simulink model "blocks"  (Simulink 6.6)
settings: Solver=FixedStepDiscrete  StartTime=0.0  StopTime=10.0  FixedStep=0.001  RelTol=1e-3
undefined symbols (not defined in the file or in its folder): ecan1_init, init_DMA0, init_DMA2, u1
libraries: simulink x11, dsPICdrivers x3
settings Model: Creator=bwmairs  LastModifiedBy=bwmairs  ProdHWDeviceType=16-bit Generic
settings OptimizationCC: InlineParams=on  OptimizeModelRefInitCode=on  LifeSpan=1
settings HardwareCC: ProdBitPerInt=16  ProdEndianess=LittleEndian  ProdWordSize=16  ProdHWDeviceType=16-bit Generic  TargetHWDeviceType=32-bit Generic
settings RTWCC: SystemTargetFile=dspic.tlc  TemplateMakefile=dspic_pic30_gcc.tmf  PostCodeGenCommand=dsPIC_Compile()  Description=Embedded Target for Microchip dsPIC (real-time)  ProcessScript=dspic_make_rtw_hook
settings CodeAppCC: IgnoreCustomStorageClasses=off
settings STFCustomTargetCC: TargetFcnLib=ansi_tfl_tmw.mat  GenFloatMathFcnCalls=ANSI_C  ModelReferenceCompliant=off  IncludeMdlTerminateFcn=off  CombineOutputUpdateFcns=on  SuppressErrorStatus=on  ERTCustomFileBanners=on  SupportContinuousTime=off  SupportNonInlinedSFcns=off  SystemTargetFile=dspic.tlc
settings ERTTargetCC: TargetFcnLib=ansi_tfl_tmw.mat  GenFloatMathFcnCalls=ANSI_C  ModelReferenceCompliant=off  IncludeMdlTerminateFcn=off  SuppressErrorStatus=on  ModelStepFunctionPrototypeControlCompliant=off  InlinedParameterPlacement=NonHierarchical  ERTSrcFileBannerTemplate=dsPIC_code_template.cgt  ERTHdrFileBannerTemplate=dsPIC_code_template.cgt  ERTDataSrcFileTemplate=dsPIC_code_template.cgt  ERTDataHdrFileTemplate=dsPIC_code_template.cgt  ERTCustomFileTemplate=dsPIC_main.tlc
settings CustomProperty: DataType=string  Value=C:\PROGRA~1\MATLAB\R2007a\rtw\bin\win32\gmake

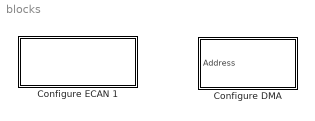
== system blocks ==
  Configure DMA : Subsystem  mask{channel=0, direction=Read, irqsel=INT0, peripheral=0, a_mode=Peripheral Indirect, mode=Continuous, half=when half of data has been moved, nullw=Null data write to peripheral, data_size=Word, batch_size=0}
      mask prompts: channel "DMA Channel"; irqsel "IRQ"; a_mode "Addressing Mode"; half "Trigger Block Transfer Interrupt"; nullw "Null Data Peripheral Write Mode"; data_size "Data Size"; batch_size "Batch Size"
      mask help: CURRENTLY HARDWIRED TO CONFIGURE DMA0!
      mask Help: Batch size - This refers to the DMAxCNT register. It consists of a 10-bit number that is 1 less than the number of requests the channel must service before the data block transfer is considered complete.
      mask StyleString: popup(0|1|2|3|4|5|6|7),popup(Read|Write),popup(INT0|IC1|OC1|IC2|OC2|TMR2|TMR3|SPI1|UART1RX|UART1TX|ADC1|ADC2|UART2RX|UART2TX|SPI2|ECAN1|ECAN2|DCI|ECAN1|ECAN2),edit,popup(Peripheral Indirect|Register Indirect|Register Indirect: Post-Increment),popup(Continuous|One-Shot|Continuous w/ Ping-Pong|One-Shot w/ Ping-Pong),popup(when half of data has been moved|when all the data has been moved),popup(Null data write to peripheral|Normal operation),popup(Word|Byte),edit
      mask Display: text(0.5,0.5,sprintf('Configure DMA%d',str2num(get_param(gcb,'channel'))),'horizontalAlignment','center','verticalAlignment','middle');
  Configure ECAN 1 : Subsystem  mask(Initialize ECAN 1){frame_setting=off, mode=--, dma_rx_chan=0, dma_tx_chan=0, baud=0, ps1=0, pd=0, ps2=0, tq=0, dma_buf_size=4 buffers, rx_bufs=[], tx_bufs=[], buf_0_tx_pri=Highest, buf_1_tx_pri=Lowest, mask_0=0, mask_0_rm=0, mask_1=0, mask_1_rm=0, mask_2=0, mask_2_rm=0, filters=[], filter_0=0, filter_0_mask=0, filter_0_exide=0, filter_0_buf=0, filter_1=0, filter_1_mask=0, filter_1_exide=0, filter_1_buf=0}
      mask prompts: frame_setting "Extended Frames (Standard if unchecked)"; dma_rx_chan "DMA Reception Channel"; dma_tx_chan "DMA Transmission Channel"; baud "Baud Rate"; ps1 "Phase Segment 1"; pd "Propagation Delay"; ps2 "Phase Segment 2"; tq "Time Quanta"; dma_buf_size "DMA Buffer Size"; rx_bufs "Reception Buffers"; tx_bufs "Transmission Buffers"; buf_0_tx_pri "Buffer 0 Transmission Priority"; buf_1_tx_pri "Buffer 1 Transmission Priority"; mask_0 "Mask 0"; mask_0_rm "Mask 0 Receive Mode"; mask_1 "Mask 1"; mask_1_rm "Mask 1 Receive Mode"; mask_2 "Mask 2"; mask_2_rm "Mask 2 Receive Mode"; filter_0 "Filter 0"; filter_0_mask "Filter 0 Mask"; filter_0_exide "Filter 0 Extended Enable"; filter_0_buf "Filter 0 Buffer"; filter_1 "Filter 1"; filter_1_mask "Filter 1 Mask"; filter_1_exide "Filter 1 Extended Enable"; filter_1_buf "Filter 1 Buffer"
      mask help: Initializes the ECAN 1 module on the dsPIC33f. Allows for configuration of almost all ECAN options to produce a usable system.
      mask StyleString: checkbox,popup(--|Normal|Loopback|Listen only|Configuration|Listen all),edit,edit,edit,edit,edit,edit,edit,popup(4 buffers|6 buffers|8 buffers|12 buffers|16 buffers|24 buffers|32 buffers),edit,edit,popup(Lowest|Low|High|Highest),popup(Lowest|Low|High|Highest),edit,popup(0|1),edit,popup(0|1),edit,popup(0|1),edit,edit,popup(--|0|1|2),popup(0|1),popup(FIFO|0|1|2|3|4|5|6|7|8|9|10|11|12|13|14),edit,popup(--|0|1|2),popup(0|1),popup(FIFO|0|1|2|3|4|5|6|7|8|9|10|11|12|13|14)
      mask CallbackString:
      | |||||tq = str2num(get_param(gcb, 'ps1')) + str2num(get_param(gcb, 'pd')) + str2num(get_param(gcb, 'ps2'));
      | set_param(gcb, 'tq', int2str(tq));|tq = str2num(get_param(gcb, 'ps1')) + str2num(get_param(gcb, 'pd')) + str2num(get_param(gcb, 'ps2'));
      | set_param(gcb, 'tq', int2str(tq));|tq = str2num(get_param(gcb, 'ps1')) + str2num(get_param(gcb, 'pd')) + str2num(get_param(gcb, 'ps2'));
      | set_param(gcb, 'tq', int2str(tq));||||filters = eval(get_param(gcb,'tx_bufs'));
      | mVisibilities = get_param(gcb,'MaskVisibilities');
      | mNames = get_param(gcb,'MaskNames');
      | for i = 1:size(mNames);
      | 	n = mNames{i};
      |     if size(n,2) > 4 && strcmp(n(1:4), 'buf_') == 1
      |         filterNumber = sscanf(n, 'buf_%d');
      |         if isempty(find(filters == filterNumber, 1)) == 0
      |              mVisibilities{i} = 'on';
      |         else
      |              mVisibilities{i} = 'off';
      |         end
      |     end
      | end
      | set_param(gcb, 'MaskVisibilities', mVisibilities);|||||||||filters = eval(get_param(gcb,'filters'));
      | mVisibilities = get_param(gcb,'MaskVisibilities');
      | mNames = get_param(gcb,'MaskNames');
      | for i = 1:size(mNames);
      | 	n = mNames{i};
      |     if size(n,2) > 7 && strcmp(n(1:7), 'filter_') == 1
      |         filterNumber = sscanf(n, 'filter_%d');
      |         if isempty(find(filters == filterNumber, 1)) == 0
      |              mVisibilities{i} = 'on';
      |         else
      |              mVisibilities{i} = 'off';
      |         end
      |     end
      | end
      | set_param(gcb, 'MaskVisibilities', mVisibilities);||||||||
      mask Display: text(0.5,0.5,'Configure ECAN1','horizontalAlignment','center','verticalAlignment','middle');

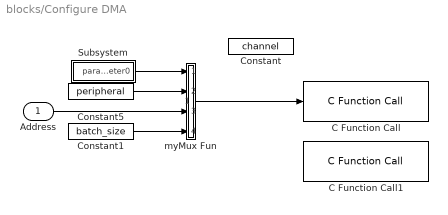
== system blocks/Configure DMA ==
  Address : Inport
  C Function Call : dsPICdrivers/OTHERS/C Function Call  Tag=dsPIC_dsPIC_CFunctionCall  fctName='init_DMA0'  INPUT_SIZE=4  INPUT1=uint16  INPUT2=--  INPUT3=--  OUTPUT_SIZE=1  OUTPUT1=--  SampleTime=inf  InputType=[ 4 ]  OutputType=[ ]  FctDeclaration=extern void init_DMA0(uint16_T* u1);  FctCall=init_DMA0(*%u1);  OrderingInOutPopup=None
  C Function Call1 : dsPICdrivers/OTHERS/C Function Call  Tag=dsPIC_dsPIC_CFunctionCall  fctName='init_DMA2'  INPUT_SIZE=4  INPUT1=uint16  INPUT2=--  INPUT3=--  OUTPUT_SIZE=1  OUTPUT1=--  SampleTime=inf  InputType=[ 4 ]  OutputType=[ ]  FctDeclaration=extern void init_DMA2(uint16_T* u1);  FctCall=init_DMA2(*%u1);  OrderingInOutPopup=None
  Constant : Constant  Value=channel
  Constant1 : Constant  Value=batch_size
  Constant5 : Constant  Value=peripheral
  Subsystem : Subsystem
  myMux Fun : Stateflow chart
  wires:
  Address/1 -> myMux Fun/3(u3)
  Subsystem/1(parameter0) -> myMux Fun/1(u1)
  Constant5/1 -> myMux Fun/2(u2)
  Constant1/1 -> myMux Fun/4(u4)
  myMux Fun/1(y) -> C Function Call/1

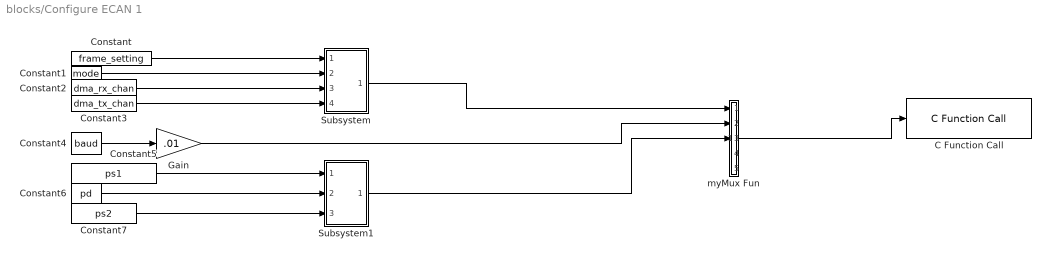
== system blocks/Configure ECAN 1 ==
  C Function Call : dsPICdrivers/OTHERS/C Function Call  Tag=dsPIC_dsPIC_CFunctionCall  fctName='ecan1_init'  INPUT_SIZE=5  INPUT1=uint16  INPUT2=--  INPUT3=--  OUTPUT_SIZE=1  OUTPUT1=--  SampleTime=inf  InputType=[ 4 ]  OutputType=[ ]  FctDeclaration=extern void ecan1_init(uint16_T* u1);  FctCall=ecan1_init(*%u1);  OrderingInOutPopup=None
  Constant : Constant  Value=frame_setting  OutDataTypeMode=uint16
  Constant1 : Constant  Value=mode  OutDataTypeMode=uint16
  Constant2 : Constant  Value=dma_rx_chan  OutDataTypeMode=uint16
  Constant3 : Constant  Value=dma_tx_chan  OutDataTypeMode=uint16
  Constant4 : Constant  Value=baud  OutDataTypeMode=uint16
  Constant5 : Constant  Value=ps1  OutDataTypeMode=uint16
  Constant6 : Constant  Value=pd  OutDataTypeMode=uint16
  Constant7 : Constant  Value=ps2  OutDataTypeMode=uint16
  Gain : Gain  Gain=.01
  Subsystem : Subsystem
  Subsystem1 : Subsystem
  myMux Fun : Stateflow chart
  wires:
  Constant4/1 -> Gain/1
  myMux Fun/1(y) -> C Function Call/1
  Constant/1 -> Subsystem/1(In1)
  Constant1/1 -> Subsystem/2(In2)
  Constant2/1 -> Subsystem/3(In3)
  Constant3/1 -> Subsystem/4(In4)
  Subsystem/1(Out1) -> myMux Fun/1(u1)
  Gain/1 -> myMux Fun/2(u2)
  Constant5/1 -> Subsystem1/1(In1)
  Constant6/1 -> Subsystem1/2(In2)
  Constant7/1 -> Subsystem1/3(In3)
  Subsystem1/1(Out1) -> myMux Fun/3(u3)

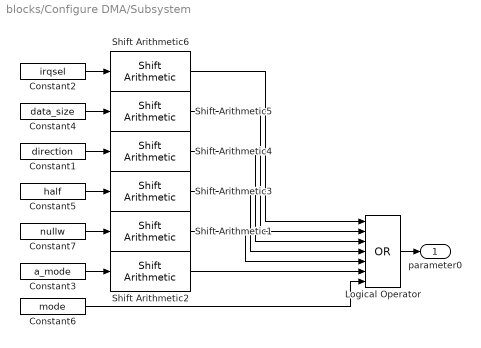
== system blocks/Configure DMA/Subsystem ==
  Constant1 : Constant  Value=direction
  Constant2 : Constant  Value=irqsel
  Constant3 : Constant  Value=a_mode
  Constant4 : Constant  Value=data_size
  Constant5 : Constant  Value=half
  Constant6 : Constant  Value=mode
  Constant7 : Constant  Value=nullw
  Logical Operator : Logic  Operator=OR  Inputs=7  AllPortsSameDT=off  OutDataTypeMode=Boolean
  Shift Arithmetic1 : simulink/Logic and Bit Operations/Shift Arithmetic  SystemSampleTime=-1  nBitShiftRight=-4  nBinPtShiftRight=0
  Shift Arithmetic2 : simulink/Logic and Bit Operations/Shift Arithmetic  SystemSampleTime=-1  nBitShiftRight=-2  nBinPtShiftRight=0
  Shift Arithmetic3 : simulink/Logic and Bit Operations/Shift Arithmetic  SystemSampleTime=-1  nBitShiftRight=-5  nBinPtShiftRight=0
  Shift Arithmetic4 : simulink/Logic and Bit Operations/Shift Arithmetic  SystemSampleTime=-1  nBitShiftRight=-6  nBinPtShiftRight=0
  Shift Arithmetic5 : simulink/Logic and Bit Operations/Shift Arithmetic  SystemSampleTime=-1  nBitShiftRight=-7  nBinPtShiftRight=0
  Shift Arithmetic6 : simulink/Logic and Bit Operations/Shift Arithmetic  SystemSampleTime=-1  nBitShiftRight=-8  nBinPtShiftRight=0
  parameter0 : Outport
  wires:
  Constant6/1 -> Logical Operator/7
  Constant3/1 -> Shift Arithmetic2/1
  Constant7/1 -> Shift Arithmetic1/1
  Logical Operator/1 -> parameter0/1
  Shift Arithmetic2/1 -> Logical Operator/6
  Shift Arithmetic1/1 -> Logical Operator/5
  Constant4/1 -> Shift Arithmetic5/1
  Constant1/1 -> Shift Arithmetic4/1
  Constant5/1 -> Shift Arithmetic3/1
  Shift Arithmetic3/1 -> Logical Operator/4
  Shift Arithmetic4/1 -> Logical Operator/3
  Shift Arithmetic5/1 -> Logical Operator/2
  Shift Arithmetic6/1 -> Logical Operator/1
  Constant2/1 -> Shift Arithmetic6/1

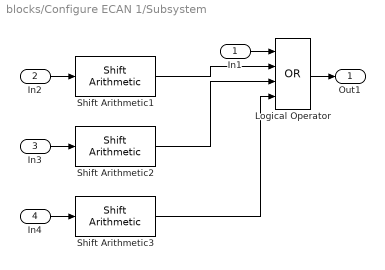
== system blocks/Configure ECAN 1/Subsystem ==
  In1 : Inport
  In2 : Inport  Port=2
  In3 : Inport  Port=3
  In4 : Inport  Port=4
  Logical Operator : Logic  Operator=OR  Inputs=4  AllPortsSameDT=off  OutDataTypeMode=Boolean
  Shift Arithmetic1 : simulink/Logic and Bit Operations/Shift Arithmetic  SystemSampleTime=-1  nBitShiftRight=-2  nBinPtShiftRight=0
  Shift Arithmetic2 : simulink/Logic and Bit Operations/Shift Arithmetic  SystemSampleTime=-1  nBitShiftRight=-5  nBinPtShiftRight=0
  Shift Arithmetic3 : simulink/Logic and Bit Operations/Shift Arithmetic  SystemSampleTime=-1  nBitShiftRight=-8  nBinPtShiftRight=0
  Out1 : Outport
  wires:
  Shift Arithmetic1/1 -> Logical Operator/2
  Shift Arithmetic2/1 -> Logical Operator/3
  Shift Arithmetic3/1 -> Logical Operator/4
  In1/1 -> Logical Operator/1
  Logical Operator/1 -> Out1/1
  In2/1 -> Shift Arithmetic1/1
  In3/1 -> Shift Arithmetic2/1
  In4/1 -> Shift Arithmetic3/1

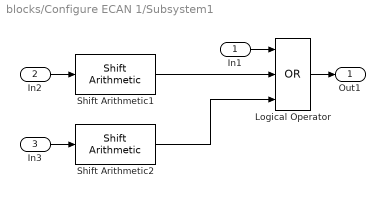
== system blocks/Configure ECAN 1/Subsystem1 ==
  In1 : Inport
  In2 : Inport  Port=2
  In3 : Inport  Port=3
  Logical Operator : Logic  Operator=OR  Inputs=3  AllPortsSameDT=off  OutDataTypeMode=Boolean
  Shift Arithmetic1 : simulink/Logic and Bit Operations/Shift Arithmetic  SystemSampleTime=-1  nBitShiftRight=-3  nBinPtShiftRight=0
  Shift Arithmetic2 : simulink/Logic and Bit Operations/Shift Arithmetic  SystemSampleTime=-1  nBitShiftRight=-6  nBinPtShiftRight=0
  Out1 : Outport
  wires:
  Shift Arithmetic1/1 -> Logical Operator/2
  Shift Arithmetic2/1 -> Logical Operator/3
  In1/1 -> Logical Operator/1
  Logical Operator/1 -> Out1/1
  In2/1 -> Shift Arithmetic1/1
  In3/1 -> Shift Arithmetic2/1

== matlab function Configure ECAN 1/myMux Fun ==
  data: u1 input inherited; y output inherited; u2 input inherited; u3 input inherited; u4 input inherited; u5 input inherited
function y = myMux3(u1, u2, u3, u4, u5)
% This block supports an embeddable subset of the MATLAB language.
% See the help menu for details. 

y = [u1(1); u2(1); u3(1); u4(1); u5(1)];

== matlab function Configure DMA/myMux Fun ==
  data: u1 input inherited; y output inherited; u2 input inherited; u3 input inherited; u4 input inherited
function y = myMux3(u1, u2, u3, u4)
% This block supports an embeddable subset of the MATLAB language.
% See the help menu for details. 

y = [u1(1); u2(1); u3(1); u4(1)];
